simulink model "part2sima"  (R2023a)
settings: Solver=VariableStepAuto  StartTime=0.0  StopTime=10.0  RelTol=1e-3
settings Model: Creator=rar4  LastModifiedBy=rar4

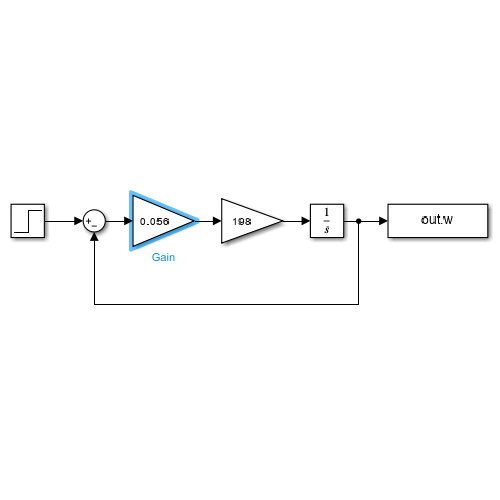
[thumbnail: Simulink's stored preview of the top-level diagram]
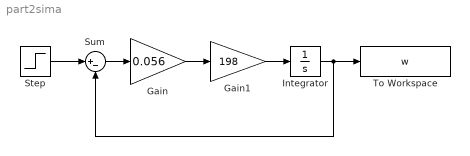
== system part2sima ==
  Gain : Gain  Gain=0.056
  Gain1 : Gain  Gain=198
  Integrator : Integrator
  Step : Step  Time=0  After=100  SampleTime=0
  Sum : Sum  Inputs=|+-
  To Workspace : ToWorkspace  VariableName=w  SampleTime=-1
  wires:
  Gain/1 -> Gain1/1
  Gain1/1 -> Integrator/1
  Integrator/1 -> Sum/2, To Workspace/1
  Step/1 -> Sum/1
  Sum/1 -> Gain/1
